simulink model "FinalProject (1)"  (R2020a)
settings: Solver=VariableStepAuto  StartTime=0.0  StopTime=10.0  RelTol=1e-3
values from neighbouring files (symbols this model uses):
  A = [0 0 1 0;0 0 0 1;0 (1/(4*Jt))*Mp^2*Lp^2*Lr*g (-1/Jt)*Br*(Jp+1/4*Mp*Lp^2) (-1/(2*Jt))*Bp*Mp*Lp*Lr;0 .5*Mp*Lp*g*(Jr+Mp*Lr^2)/Jt (1/(2*Jt))*Mp*Lp*Lr*Br (-1/Jt)*Bp*(Jr+Mp*Lp^2)]    [StateSpaceRep (4).m]
  B = Kg*kt*B/Rm    [StateSpaceRep (4).m]
  C = eye(2,4)    [StateSpaceRep (4).m]
  D = zeros(2,1)    [StateSpaceRep (4).m]
  Er = Ep    (= 0.41985819)    [StateSpaceRep (4).m]
  eta_g = 0.70    (= 0.7)    [StateSpaceRep (4).m]
  eta_m = 0.90    (= 0.9)    [StateSpaceRep (4).m]
  g = 9.81    [StateSpaceRep (4).m]
  Jp = .8    (= 0.8)    [StateSpaceRep (4).m]
  K = acker(A, B, poles)    [StateSpaceRep (4).m]
  K_amp = 2.5    [StateSpaceRep (4).m]
  Kg = .9    (= 0.9)    [StateSpaceRep (4).m]
  km = .03    (= 0.03)    [StateSpaceRep (4).m]
  kt = 0.00768    [StateSpaceRep (4).m]
  Lp = .337    (= 0.337)    [StateSpaceRep (4).m]
  Lr = .216    (= 0.216)    [StateSpaceRep (4).m]
  Mp = .127    (= 0.127)    [StateSpaceRep (4).m]
  Mr = .125    (= 0.125)    [StateSpaceRep (4).m]
  mu = 2.3    [StateSpaceRep (4).m]
  Rm = 2.6    [StateSpaceRep (4).m]
undefined symbols (not defined in the file or in its folder): epsilon
libraries: simulink x2, aerolibconvert2 x1, dspsrcs4 x1, dspsnks4 x1
settings Model: Creator=victo  LastModifiedBy=victo

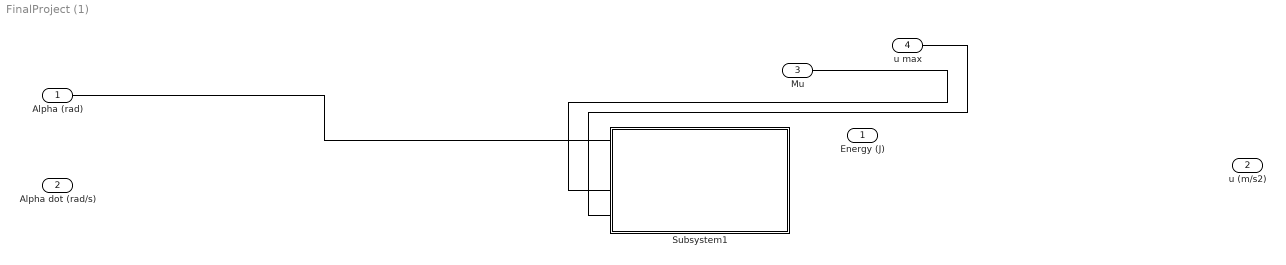
== system FinalProject (1) ==
  Alpha (rad) : Inport
  Alpha dot (rad/s) : Inport  Port=2
  Mu : Inport  Port=3
  u max : Inport  Port=4
  Subsystem1 : Subsystem
  Energy (J) : Outport
  u (m/s2) : Outport  Port=2
  wires:
  u max/1 -> ?
  Mu/1 -> ?
  Alpha (rad)/1 -> ?
  ? -> Energy (J)/1
  ? -> u (m/s2)/1

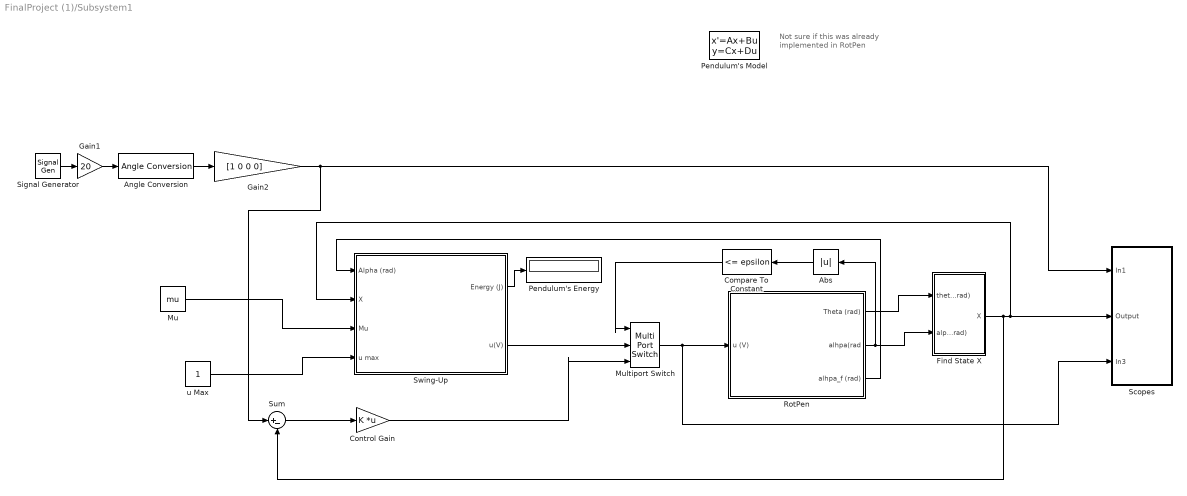
== system FinalProject (1)/Subsystem1 ==
  note: Not sure if this was already implemented in RotPen
  Abs : Abs
  Angle Conversion : aerolibconvert2/Angle Conversion  IU=deg  OU=rad
  Compare To Constant : simulink/Logic and Bit Operations/Compare To Constant  relop=<=  const=epsilon  OutDataTypeStr=boolean
  Control Gain : Gain  Gain=K  Multiplication=Matrix(K*u)
  Find State X : Subsystem
  Gain1 : Gain  Gain=20
  Gain2 : Gain  Gain=[1 0 0 0]
  Mu : Constant  Value=mu
  Multiport Switch : MultiPortSwitch  Inputs=2
  Pendulum's Energy : Display
  Pendulum's Model : StateSpace  A=A  B=B  C=C  D=D  InitialCondition=0
  RotPen : Subsystem
  Scopes : Subsystem
  Signal Generator : SignalGenerator  Units=rad/sec
  Sum : Sum  Inputs=|+-
  Swing-Up : Subsystem
  u Max : Constant
  wires:
  Swing-Up/1(Energy (J)) -> Pendulum's Energy/1
  Signal Generator/1 -> Gain1/1
  Gain1/1 -> Angle Conversion/1
  Angle Conversion/1 -> Gain2/1
  Gain2/1 -> Scopes/1(In1), Sum/1
  RotPen/3(alhpa_f (rad)) -> Swing-Up/1(Alpha (rad))
  Sum/1 -> Control Gain/1
  Find State X/1(X) -> Sum/2, Swing-Up/2(X), Scopes/2(Output)
  RotPen/2(alhpa(rad) -> Abs/1, Find State X/2(alpha (rad))
  RotPen/1(Theta (rad)) -> Find State X/1(theta (rad))
  Swing-Up/2(u(V)) -> Multiport Switch/2
  Multiport Switch/1 -> Scopes/3(In3), RotPen/1(u (V))
  Control Gain/1 -> Multiport Switch/3
  Abs/1 -> Compare To Constant/1
  Compare To Constant/1 -> Multiport Switch/1
  u Max/1 -> Swing-Up/4(u max)
  Mu/1 -> Swing-Up/3(Mu)

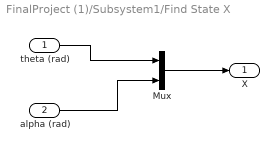
== system FinalProject (1)/Subsystem1/Find State X ==
  theta (rad) : Inport
  alpha (rad) : Inport  Port=2
  Mux : Mux  Inputs=2
  X : Outport
  wires:
  Mux/1 -> X/1
  theta (rad)/1 -> Mux/1
  alpha (rad)/1 -> Mux/2

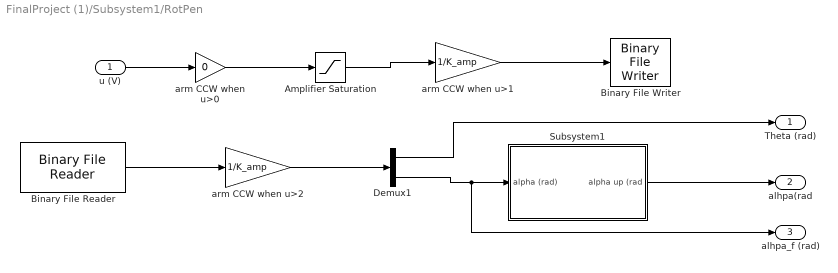
== system FinalProject (1)/Subsystem1/RotPen ==
  u (V) : Inport
  Amplifier Saturation : Saturate
  Binary File Reader : dspsrcs4/Binary File Reader  Filename=Untitled.bin  HeaderStructure=struct([])  DataType=double  SamplesPerFrame=1024  IsDataComplex=off  NumChannels=1  OutputEOF=off  SampleTime=1  SimulateUsing=Code generation
      settings: SourceProductBaseCode=DS
  Binary File Writer : dspsnks4/Binary File Writer  Filename=Untitled.bin  HeaderStructure=struct([])  SimulateUsing=Code generation
      settings: SourceProductBaseCode=DS
  Demux1 : Demux  Outputs=2
  Subsystem1 : Subsystem
  arm CCW when u>0 : Gain  Gain=0
  arm CCW when u>1 : Gain  Gain=1/K_amp
  arm CCW when u>2 : Gain  Gain=1/K_amp
  Theta (rad) : Outport
  alhpa(rad : Outport  Port=2
  alhpa_f (rad) : Outport  Port=3
  wires:
  arm CCW when u>1/1 -> Binary File Writer/1
  arm CCW when u>0/1 -> Amplifier Saturation/1
  Binary File Reader/1 -> arm CCW when u>2/1
  Demux1/1 -> Theta (rad)/1
  u (V)/1 -> arm CCW when u>0/1
  Amplifier Saturation/1 -> arm CCW when u>1/1
  Demux1/2 -> alhpa_f (rad)/1, Subsystem1/1(alpha (rad))
  arm CCW when u>2/1 -> Demux1/1
  Subsystem1/1(alpha up (rad) -> alhpa(rad/1

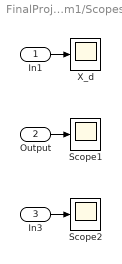
== system FinalProject (1)/Subsystem1/Scopes ==
  In1 : Inport
  Output : Inport  Port=2
  In3 : Inport  Port=3
  Scope1 : Scope
  Scope2 : Scope
  X_d : Scope
  wires:
  In1/1 -> X_d/1
  In3/1 -> Scope2/1
  Output/1 -> Scope1/1

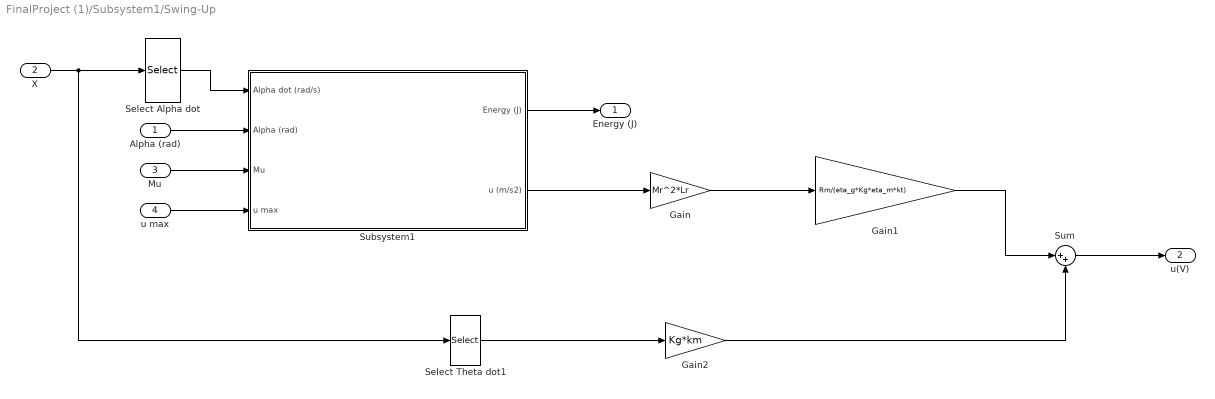
== system FinalProject (1)/Subsystem1/Swing-Up ==
  Alpha (rad) : Inport
  X : Inport  Port=2
  Mu : Inport  Port=3
  u max : Inport  Port=4
  Gain : Gain  Gain=Mr^2*Lr
  Gain1 : Gain  Gain=Rm/(eta_g*Kg*eta_m*kt)
  Gain2 : Gain  Gain=Kg*km
  Select Alpha dot : Selector  InputPortWidth=3  IndexOptions=Index vector (dialog)  Indices=[1 3]  OutputSizes=1
  Select Theta dot1 : Selector  InputPortWidth=3  IndexOptions=Index vector (dialog)  Indices=[1 3]  OutputSizes=1
  Subsystem1 : Subsystem
  Sum : Sum  Inputs=|++
  Energy (J) : Outport
  u(V) : Outport  Port=2
  wires:
  X/1 -> Select Theta dot1/1, Select Alpha dot/1
  Subsystem1/2(u (m/s2)) -> Gain/1
  Gain1/1 -> Sum/1
  Sum/1 -> u(V)/1
  Subsystem1/1(Energy (J)) -> Energy (J)/1
  Mu/1 -> Subsystem1/3(Mu)
  Gain/1 -> Gain1/1
  u max/1 -> Subsystem1/4(u max)
  Alpha (rad)/1 -> Subsystem1/2(Alpha (rad))
  Gain2/1 -> Sum/2
  Select Theta dot1/1 -> Gain2/1
  Select Alpha dot/1 -> Subsystem1/1(Alpha dot (rad/s))

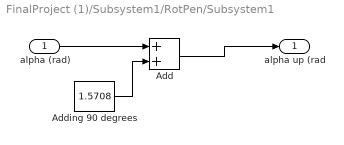
== system FinalProject (1)/Subsystem1/RotPen/Subsystem1 ==
  alpha (rad) : Inport
  Add : Sum
  Adding 90 degrees : Constant  Value=1.5708
  alpha up (rad : Outport
  wires:
  alpha (rad)/1 -> Add/1
  Adding 90 degrees/1 -> Add/2
  Add/1 -> alpha up (rad/1

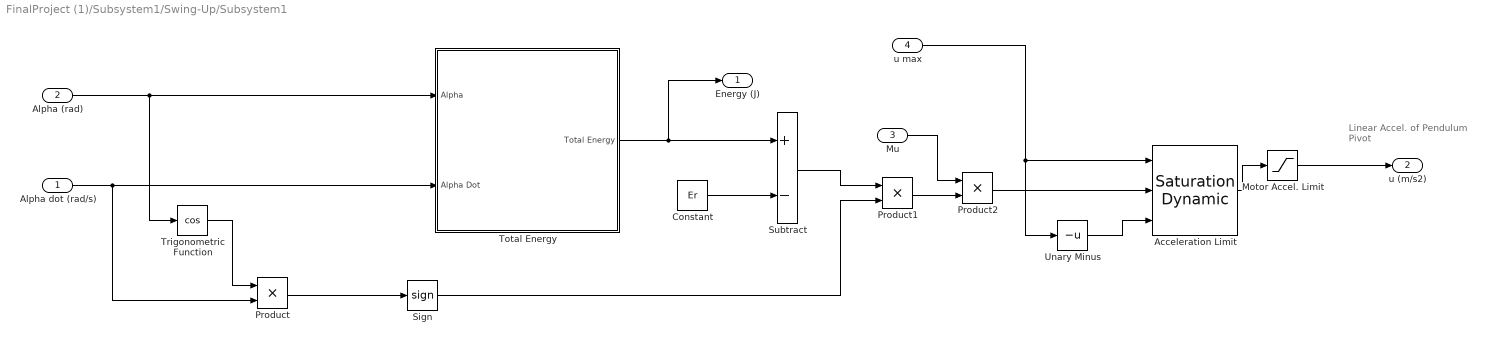
== system FinalProject (1)/Subsystem1/Swing-Up/Subsystem1 ==
  note: Linear Accel. of Pendulum Pivot
  Alpha dot (rad/s) : Inport
  Alpha (rad) : Inport  Port=2
  Mu : Inport  Port=3
  u max : Inport  Port=4
  Acceleration Limit : simulink/Discontinuities/Saturation Dynamic  OutMin=[]  OutMax=[]  OutDataTypeStr=Inherit: Same as second input  OutDataType=fixdt(1, 16)  OutScaling=2^-10  DoSatur=off
  Constant : Constant  Value=Er
  Motor Accel. Limit : Saturate
  Product : Product
  Product1 : Product
  Product2 : Product
  Sign : Signum
  Subtract : Sum  Inputs=+-
  Total Energy : Subsystem
  Trigonometric Function : Trigonometry  Operator=cos
  Unary Minus : UnaryMinus
  Energy (J) : Outport
  u (m/s2) : Outport  Port=2
  wires:
  u max/1 -> Acceleration Limit/1, Unary Minus/1
  Product2/1 -> Acceleration Limit/2
  Motor Accel. Limit/1 -> u (m/s2)/1
  Alpha (rad)/1 -> Trigonometric Function/1, Total Energy/1("Alpha ")
  Alpha dot (rad/s)/1 -> Product/2, Total Energy/2(Alpha Dot)
  Unary Minus/1 -> Acceleration Limit/3
  Mu/1 -> Product2/1
  Product1/1 -> Product2/2
  Sign/1 -> Product1/2
  Total Energy/1(Total Energy) -> Energy (J)/1, Subtract/1
  Product/1 -> Sign/1
  Trigonometric Function/1 -> Product/1
  Acceleration Limit/1 -> Motor Accel. Limit/1
  Constant/1 -> Subtract/2
  Subtract/1 -> Product1/1

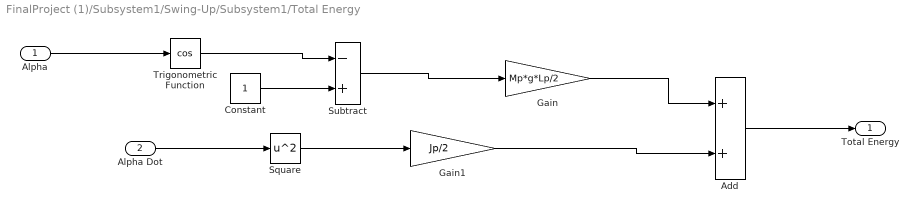
== system FinalProject (1)/Subsystem1/Swing-Up/Subsystem1/Total Energy ==
  "Alpha " : Inport
  Alpha Dot : Inport  Port=2
  Add : Sum
  Constant : Constant
  Gain : Gain  Gain=Mp*g*Lp/2
  Gain1 : Gain  Gain=Jp/2
  Square : Math  Operator=square  SaturateOnIntegerOverflow=on
  Subtract : Sum  Inputs=-+
  Trigonometric Function : Trigonometry  Operator=cos
  Total Energy : Outport
  wires:
  Subtract/1 -> Gain/1
  Gain/1 -> Add/1
  Square/1 -> Gain1/1
  Trigonometric Function/1 -> Subtract/1
  Constant/1 -> Subtract/2
  Gain1/1 -> Add/2
  "Alpha "/1 -> Trigonometric Function/1
  Add/1 -> Total Energy/1
  Alpha Dot/1 -> Square/1
